simulink model "ScalarModel"  (R2022b)
settings: Solver=ode45  StartTime=0.0  StopTime=30  RelTol=1e-3
values from neighbouring files (symbols this model uses):
  alpha0 = 0    [Run_Both_Model.m]    (also in Run_Deadzone.m; Run_ScalarModel.m; Slicing.m; UniCenterMRAC.m)
  ar = -20    [Run_Both_Model.m]    (also in Run_Deadzone.m; Run_Project1i_haoran9.m; Run_ScalarModel.m; Slicing.m)
  astar = -10    [Run_Both_Model.m]    (also in Run_Deadzone.m; Run_Project1i_haoran9.m; Run_ScalarModel.m; Slicing.m)
  basiscenter = linspace(-10,10,N)'    [Run_Both_Model.m]    (also in Run_Deadzone.m; Run_ScalarModel.m; Slicing.m; runClassicMRAC.m = linspace(-10,10,N))
  beta0 = 0    [Run_Both_Model.m]    (also in Run_Deadzone.m; Run_ScalarModel.m; Slicing.m; UniCenterMRAC.m)
  br = 20    [Run_Both_Model.m]    (also in Run_Deadzone.m; Run_Project1i_haoran9.m; Run_ScalarModel.m; Slicing.m)
  bstar = +10    (= 10)    [Run_Both_Model.m]    (also in Run_Deadzone.m; Run_Project1i_haoran9.m; Run_ScalarModel.m; Slicing.m)
  ga = 10    [Run_Both_Model.m]    (also in Run_Deadzone.m; Run_ScalarModel.m; Slicing.m; UniCenterMRAC.m = 0)
  gb = 10    [Run_Both_Model.m]    (also in Run_Deadzone.m; Run_ScalarModel.m; Slicing.m; UniCenterMRAC.m = 0)
  gf = 10    [Run_Both_Model.m]    (also in Run_Deadzone.m; Run_ScalarModel.m; Slicing.m; UniCenterMRAC.m = 1)
  hype = 1/(2*2^2)    (= 0.125)    [Run_Both_Model.m]    (also in Run_Deadzone.m; Run_ScalarModel.m; Slicing.m)
  inv_k_xi_xi3m = inv(k_xi_xi3m)    [Run_Both_Model.m]    (also in Run_Deadzone.m; Run_ScalarModel.m; Slicing.m)
  inv_k_xi_xi5m = inv(k_xi_xi5m)    [Run_Both_Model.m]    (also in Run_Deadzone.m; Run_ScalarModel.m; Slicing.m)
  inv_k_xi_xie = inv(k_xi_xie)    [Run_Both_Model.m]    (also in Run_Deadzone.m; Run_ScalarModel.m; Slicing.m)
  l = 2    [Run_Both_Model.m]    (also in Run_Deadzone.m; Run_ScalarModel.m; Slicing.m; runCompareBasisMRAC.m = 1./diag(L2))
  sig = 2    [Run_Both_Model.m]    (also in Run_Deadzone.m; Run_ScalarModel.m; Slicing.m; runMatern_MRAC.m)
  sigma = 0.1    [Run_Both_Model.m]    (also in Run_Deadzone.m; Run_Project1i_haoran9.m; Run_ScalarModel.m; Slicing.m)
  x0 = 0    [Run_Both_Model.m]    (also in Run_Deadzone.m; Run_Project1i_haoran9.m = 1; Run_ScalarModel.m; Slicing.m = 5)
  xr0 = 0    [Run_Both_Model.m]    (also in Run_Deadzone.m; Run_Project1i_haoran9.m; Run_ScalarModel.m; Slicing.m)
libraries: simulink x5
settings Model: Creator=owned  LastModifiedBy=Nathan
settings SolverCC: AlgebraicLoopSolver=TrustRegion
settings DebuggingCC: UnconnectedInputMsg=warning  UnconnectedOutputMsg=warning  UnconnectedLineMsg=warning  SFMachineParentedDataDiag=warning
settings ModelReferenceCC: EnableRefExpFcnMdlSchedulingChecks=on
settings RTWCC: DLArmComputeVersion=19.05

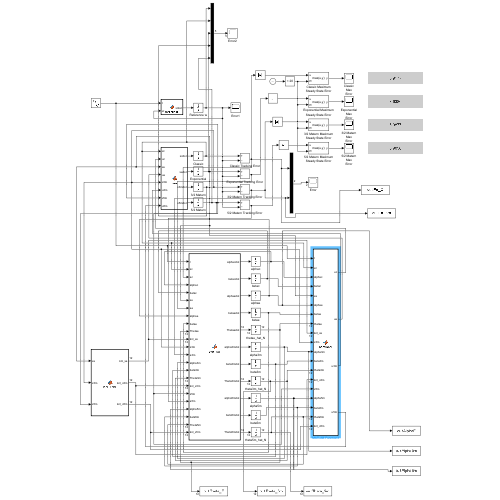
[thumbnail: Simulink's stored preview of the top-level diagram]
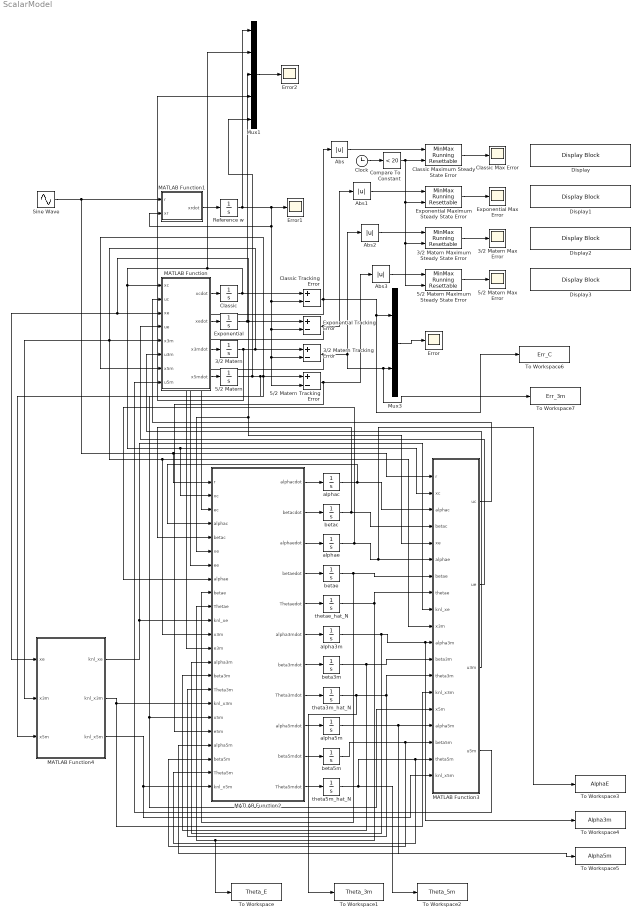
== system ScalarModel ==
  3/2 Matern : Integrator  InitialCondition=x0
  3/2 Matern Max Error : Scope
  3/2 Matern Maximum Steady State Error : simulink/Math Operations/MinMax Running Resettable  Function=max  vinit=0.0
  3/2 Matern Tracking Error : Sum  Inputs=+-
  5/2 Matern : Integrator  InitialCondition=x0
  5/2 Matern Max Error : Scope
  5/2 Matern Maximum Steady State Error : simulink/Math Operations/MinMax Running Resettable  Function=max  vinit=0.0
  5/2 Matern Tracking Error : Sum  Inputs=+-
  Abs{,1..3} (4 alike) : Abs  SaturateOnIntegerOverflow=off
  Classic : Integrator  InitialCondition=x0
  Classic Max Error : Scope
  Classic Maximum Steady State Error : simulink/Math Operations/MinMax Running Resettable  Function=max  vinit=0.0
  Classic Tracking Error : Sum  Inputs=+-
  Clock : Clock
  Compare To Constant : simulink/Logic and Bit Operations/Compare To Constant  relop=<  const=20  OutDataTypeStr=boolean
  Display{,1..3} (4 alike) : DisplayBlock  LabelPosition=Hide  Transparency=1
  Error : Scope
  Error1 : Scope
  Error2 : Scope
  Exponential : Integrator  InitialCondition=x0
  Exponential Max Error : Scope
  Exponential Maximum Steady State Error : simulink/Math Operations/MinMax Running Resettable  Function=max  vinit=0.0
  Exponential Tracking Error : Sum  Inputs=+-
  MATLAB Function : MATLAB Function  TreatAsAtomicUnit=on
  MATLAB Function1 : MATLAB Function  TreatAsAtomicUnit=on
  MATLAB Function2 : MATLAB Function  TreatAsAtomicUnit=on
  MATLAB Function3 : MATLAB Function  TreatAsAtomicUnit=on
  MATLAB Function4 : MATLAB Function  TreatAsAtomicUnit=on
  Mux1 : Mux  Inputs=5
  Mux3 : Mux  Inputs=2
  Reference w : Integrator  InitialCondition=xr0
  Sine Wave : Sin  Amplitude=10  Frequency=2  SampleTime=0
  To Workspace : ToWorkspace  VariableName=Theta_E  SaveFormat=Timeseries  SampleTime=-1
  To Workspace1 : ToWorkspace  VariableName=Theta_3m  SaveFormat=Timeseries  SampleTime=-1
  To Workspace2 : ToWorkspace  VariableName=Theta_5m  SaveFormat=Timeseries  SampleTime=-1
  To Workspace3 : ToWorkspace  VariableName=AlphaE  SaveFormat=Timeseries  SampleTime=-1
  To Workspace4 : ToWorkspace  VariableName=Alpha3m  SaveFormat=Timeseries  SampleTime=-1
  To Workspace5 : ToWorkspace  VariableName=Alpha5m  SaveFormat=Timeseries  SampleTime=-1
  To Workspace6 : ToWorkspace  VariableName=Err_C  SaveFormat=Timeseries  SampleTime=-1
  To Workspace7 : ToWorkspace  VariableName=Err_3m  SaveFormat=Timeseries  SampleTime=-1
  alpha3m : Integrator  InitialCondition=alpha0
  alpha5m : Integrator  InitialCondition=alpha0
  alphac : Integrator  InitialCondition=alpha0
  alphae : Integrator  InitialCondition=alpha0
  beta3m : Integrator  InitialCondition=beta0
  beta5m : Integrator  InitialCondition=beta0
  betac : Integrator  InitialCondition=beta0
  betae : Integrator  InitialCondition=beta0
  theta3m_hat_N : Integrator
  theta5m_hat_N : Integrator
  thetae_hat_N : Integrator
  wires:
  MATLAB Function/1(xcdot) -> Classic/1
  Classic/1 -> Mux1/2, MATLAB Function3/2(xc), MATLAB Function2/2(xc), MATLAB Function/1(xc), Classic Tracking Error/1
  Sine Wave/1 -> MATLAB Function1/1(r), MATLAB Function2/1(r), MATLAB Function3/1(r)
  MATLAB Function1/1(xrdot) -> Reference w/1
  Reference w/1 -> Error1/1, Classic Tracking Error/2, Exponential Tracking Error/2, 3/2 Matern Tracking Error/2, 5/2 Matern Tracking Error/2, MATLAB Function1/2(xr), Mux1/1
  Classic Tracking Error/1 -> MATLAB Function2/3(ec), To Workspace6/1, Mux3/1, Abs/1
  Mux3/1 -> Error/1
  MATLAB Function/2(xedot) -> Exponential/1
  MATLAB Function/3(x3mdot) -> 3/2 Matern/1
  MATLAB Function/4(x5mdot) -> 5/2 Matern/1
  5/2 Matern/1 -> Mux1/5, MATLAB Function4/3(x5m), MATLAB Function2/18(x5m), MATLAB Function3/15(x5m), MATLAB Function/7(x5m), 5/2 Matern Tracking Error/1
  3/2 Matern/1 -> Mux1/4, 3/2 Matern Tracking Error/1, MATLAB Function3/10(x3m), MATLAB Function2/12(x3m), MATLAB Function/5(x3m), MATLAB Function4/2(x3m)
  Exponential/1 -> Mux1/3, MATLAB Function3/5(xe), MATLAB Function2/6(xe), MATLAB Function4/1(xe), MATLAB Function/3(xe), Exponential Tracking Error/1
  Exponential Tracking Error/1 -> Abs1/1, MATLAB Function2/7(ee)
  3/2 Matern Tracking Error/1 -> To Workspace7/1, Mux3/2, Abs2/1, MATLAB Function2/13(e3m)
  5/2 Matern Tracking Error/1 -> Abs3/1, MATLAB Function2/19(e5m)
  MATLAB Function2/1(alphacdot) -> alphac/1
  MATLAB Function2/2(betacdot) -> betac/1
  MATLAB Function2/3(alphaedot) -> alphae/1
  MATLAB Function2/4(betaedot) -> betae/1
  MATLAB Function2/5(Thetaedot) -> thetae_hat_N/1
  MATLAB Function2/6(alpha3mdot) -> alpha3m/1
  MATLAB Function2/7(beta3mdot) -> beta3m/1
  MATLAB Function2/8(Theta3mdot) -> theta3m_hat_N/1
  MATLAB Function2/9(alpha5mdot) -> alpha5m/1
  MATLAB Function2/10(beta5mdot) -> beta5m/1
  MATLAB Function2/11(Theta5mdot) -> theta5m_hat_N/1
  MATLAB Function4/1(knl_xe) -> MATLAB Function2/11(knl_xe), MATLAB Function3/9(knl_xe)
  MATLAB Function4/2(knl_x3m) -> MATLAB Function2/17(knl_x3m), MATLAB Function3/14(knl_x3m)
  MATLAB Function4/3(knl_x5m) -> MATLAB Function2/23(knl_x5m), MATLAB Function3/19(knl_x5m)
  alphac/1 -> MATLAB Function2/4(alphac), MATLAB Function3/3(alphac)
  betac/1 -> MATLAB Function2/5(betac), MATLAB Function3/4(betac)
  alphae/1 -> To Workspace3/1, MATLAB Function3/6(alphae), MATLAB Function2/8(alphae)
  betae/1 -> MATLAB Function2/9(betae), MATLAB Function3/7(betae)
  thetae_hat_N/1 -> To Workspace/1, MATLAB Function2/10(Thetae), MATLAB Function3/8(thetae)
  alpha3m/1 -> To Workspace4/1, MATLAB Function3/11(alpha3m), MATLAB Function2/14(alpha3m)
  beta3m/1 -> MATLAB Function3/12(beta3m), MATLAB Function2/15(beta3m)
  theta3m_hat_N/1 -> To Workspace1/1, MATLAB Function2/16(Theta3m), MATLAB Function3/13(theta3m)
  alpha5m/1 -> To Workspace5/1, MATLAB Function3/16(alpha5m), MATLAB Function2/20(alpha5m)
  beta5m/1 -> MATLAB Function2/21(beta5m), MATLAB Function3/17(beta5m)
  theta5m_hat_N/1 -> To Workspace2/1, MATLAB Function2/22(Theta5m), MATLAB Function3/18(theta5m)
  MATLAB Function3/1(uc) -> MATLAB Function/2(uc)
  MATLAB Function3/2(ue) -> MATLAB Function/4(ue)
  MATLAB Function3/3(u3m) -> MATLAB Function/6(u3m)
  MATLAB Function3/4(u5m) -> MATLAB Function/8(u5m)
  Clock/1 -> Compare To Constant/1
  Compare To Constant/1 -> 5/2 Matern Maximum Steady State Error/2, 3/2 Matern Maximum Steady State Error/2, Exponential Maximum Steady State Error/2, Classic Maximum Steady State Error/2
  Classic Maximum Steady State Error/1 -> Classic Max Error/1
  Exponential Maximum Steady State Error/1 -> Exponential Max Error/1
  3/2 Matern Maximum Steady State Error/1 -> 3/2 Matern Max Error/1
  5/2 Matern Maximum Steady State Error/1 -> 5/2 Matern Max Error/1
  Abs/1 -> Classic Maximum Steady State Error/1
  Abs1/1 -> Exponential Maximum Steady State Error/1
  Abs2/1 -> 3/2 Matern Maximum Steady State Error/1
  Abs3/1 -> 5/2 Matern Maximum Steady State Error/1
  Mux1/1 -> Error2/1

== matlab function ScalarModel/MATLAB Function3 ==
  data: r input; xc input; alphac input; uc output size=1; betac input; xe input; alphae input; betae input; thetae input; knl_xe input; x3m input; alpha3m input; beta3m input; theta3m input; knl_x3m input; x5m input; alpha5m input; beta5m input; theta5m input; knl_x5m input; ue output size=1; u3m output size=1; u5m output size=1
function [uc, ue, u3m, u5m]= controller(r, xc,alphac,betac,...
    xe,alphae,betae, thetae,knl_xe,x3m,alpha3m,beta3m, theta3m,knl_x3m...
    , x5m,alpha5m,beta5m, theta5m,knl_x5m)

% Classic
uc = alphac*xc+betac*r;
% Exponential
ue = alphae*xe+betae*r-thetae'*knl_xe;
% ue = betae*r-thetae'*knl_xe;
% Matern 3/2
u3m = alpha3m*x3m+beta3m*r-theta3m'*knl_x3m;
% u3m = beta3m*r-theta3m'*knl_x3m;
% Matern 5/2
u5m = alpha5m*x5m+beta5m*r-theta5m'*knl_x5m;
% u5m = beta5m*r-theta5m'*knl_x5m;

== matlab function ScalarModel/MATLAB Function4 ==
  data: xe input; x3m input; x5m input; knl_xe output; basiscenter parameter; hype parameter; sig parameter; l parameter; knl_x3m output; knl_x5m output
function [knl_xe,knl_x3m,knl_x5m] = Knl_Eval(xe,x3m,x5m,basiscenter,hype,sig,l)

knlfune=@(x,bsc) exp(-hype*(x-bsc).^2);
knlfun3m=@(x,bsc) sig^2.*(1+sqrt(3)./l.*abs(x-bsc)).*exp(-sqrt(3).*abs(x-bsc)./l);
knlfun5m=@(x,bsc) sig^2.*(1+sqrt(5)/l.*abs(x-bsc)+5/(3*l^2).*abs(x-bsc).^2).*exp(-sqrt(5).*abs(x-bsc)./l);
knl_xe=zeros(length(basiscenter),1);
knl_x3m=zeros(length(basiscenter),1);
knl_x5m=zeros(length(basiscenter),1);
for i=1:length(basiscenter)
    knl_xe(i)=knlfune(xe,basiscenter(i));
end
for i=1:length(basiscenter)
    knl_x3m(i)=knlfun3m(x3m,basiscenter(i));
end
for i=1:length(basiscenter)
    knl_x5m(i)=knlfun5m(x5m,basiscenter(i));
end

== matlab function ScalarModel/MATLAB Function1 ==
  data: r input; xr input; xrdot output; ar parameter; br parameter
function xrdot = reference(r,xr,ar, br)

xrdot = ar*xr+br*r;

== matlab function ScalarModel/MATLAB Function ==
  data: xc input; uc input; xe input; ue input; x3m input; u3m input; x5m input; u5m input; xcdot output; astar parameter; bstar parameter; xedot output; x3mdot output; x5mdot output
function [xcdot,xedot,x3mdot,x5mdot] = plant(xc,uc,xe,ue,x3m,u3m,x5m,u5m,astar, bstar)

xcdot = astar*xc+bstar*(uc+10*tanh(xc));
xedot = astar*xe+bstar*(ue+10*tanh(xe));
x3mdot = astar*x3m+bstar*(u3m+10*tanh(x3m));
x5mdot = astar*x5m+bstar*(u5m+10*tanh(x5m));

== matlab function ScalarModel/MATLAB Function2 ==
  data: ga parameter; alphacdot output size=1; betacdot output size=1; gb parameter; gf parameter; alphaedot output size=1; sigma parameter; betaedot output size=1; Thetaedot output size=N; alpha3mdot output size=1; beta3mdot output size=1; Theta3mdot output size=N; alpha5mdot output size=1; beta5mdot output size=1; Theta5mdot output size=N; r input; xc input; ec input; alphac input; betac input; xe input; ee input; alphae input; betae input; Thetae input; knl_xe input; x3m input; e3m input; alpha3m input; beta3m input; Theta3m input; knl_x3m input; x5m input; e5m input; alpha5m input; beta5m input; Theta5m input; knl_x5m input; inv_k_xi_xie parameter; inv_k_xi_xi3m parameter; inv_k_xi_xi5m parameter
function [alphacdot,betacdot,alphaedot,betaedot,Thetaedot...
    ,alpha3mdot,beta3mdot,Theta3mdot,alpha5mdot,beta5mdot,Theta5mdot]...
    = evo_law(ga, gb, gf, sigma, r, xc, ec, alphac, betac, xe, ee, alphae, betae,Thetae,...
    knl_xe,x3m, e3m,alpha3m, beta3m,Theta3m, knl_x3m,...
    x5m, e5m, alpha5m, beta5m,Theta5m, knl_x5m, inv_k_xi_xie, inv_k_xi_xi3m, inv_k_xi_xi5m)
%% Classic Case
alphacdot=-ga*xc*ec-sigma*alphac;
betacdot=-gb*r*ec-sigma*betac;
%% Exponential Case
alphaedot=-ga*xe*ee-sigma*alphae;
betaedot=-gb*r*ee-sigma*betae;
Thetaedot=gf*inv_k_xi_xie*knl_xe*ee-sigma*Thetae;
%% Matern 3/2 Case
alpha3mdot=-ga*x3m*e3m-sigma*alpha3m;
beta3mdot=-gb*r*e3m-sigma*beta3m;
Theta3mdot=gf*inv_k_xi_xi3m*knl_x3m*e3m-sigma*Theta3m;
%% Matern 5/2 Case
alpha5mdot=-ga*x5m*e5m-sigma*alpha5m;
beta5mdot=-gb*r*e5m-sigma*beta5m;
Theta5mdot=gf*inv_k_xi_xi5m*knl_x5m*e5m-sigma*Theta5m;
